simulink model "external_state_machine"  (R2021a)
settings: Solver=FixedStepDiscrete  StartTime=0.0  StopTime=3*t_ADC  RelTol=1e-3
values from neighbouring files (symbols this model uses):
  t_ADC = 1/f_ADC    (= 1e-05)    [uz_6ph_pu_vsd_voltages_init.m]    (also in uz_mpc_6ph_init.m; uz_mpc_6ph_state_machine_init.m; uz_typeconv_init.m)
  t_clock = 1/f_clock    (= 1e-08)    [uz_6ph_pu_vsd_voltages_init.m]    (also in uz_mpc_6ph_init.m; uz_mpc_6ph_state_machine_init.m; uz_typeconv_init.m)
libraries: simulink x5, hdlsllib x1
settings Model: DataTypeOverride=Off  Creator=micha  LastModifiedBy=micha
settings SolverCC: AlgebraicLoopSolver=TrustRegion
settings DataIOCC: LimitDataPoints=on  SaveOutput=off  SaveTime=off
settings OptimizationCC: BlockReduction=off  ConditionallyExecuteInputs=off  DefaultParameterBehavior=Inlined  LifeSpan=inf
settings DebuggingCC: AlgebraicLoopMsg=error  SingleTaskRateTransMsg=error  AllowSymbolicDim=off  StrictBusMsg=ErrorOnBusTreatedAsVector  SFUnexpectedBacktrackingDiag=warning  SFNoUnconditionalDefaultTransitionDiag=warning  SFExecutionAtInitializationDiag=none  SFMachineParentedDataDiag=warning  ArithmeticOperatorsInVariantConditions=warning
settings HardwareCC: ProdBitPerPointer=32  ProdBitPerSizeT=32  ProdBitPerPtrDiffT=32  ProdLargestAtomicFloat=None  ProdIntDivRoundTo=Undefined  ProdEndianess=Unspecified  ProdWordSize=32  ProdHWDeviceType=ASIC/FPGA->ASIC/FPGA  ProdEqTarget=off
settings SFSimCC: SimUseLocalCustomCode=off  CustomCodeUndefinedFunction=UseInterfaceOnly
settings RTWCC: RTWUseLocalCustomCode=off
settings CodeAppCC: StateflowObjectComments=on
settings GRTTargetCC: TargetLangStandard=C89/C90 (ANSI)
settings ConfigComp: CovScope=ReferencedModels  CovMetricSettings=dw  CovSaveCumulativeToWorkspaceVar=on  CovSaveSingleToWorkspaceVar=on  CovExternalEMLEnable=off  CovSFcnEnable=off

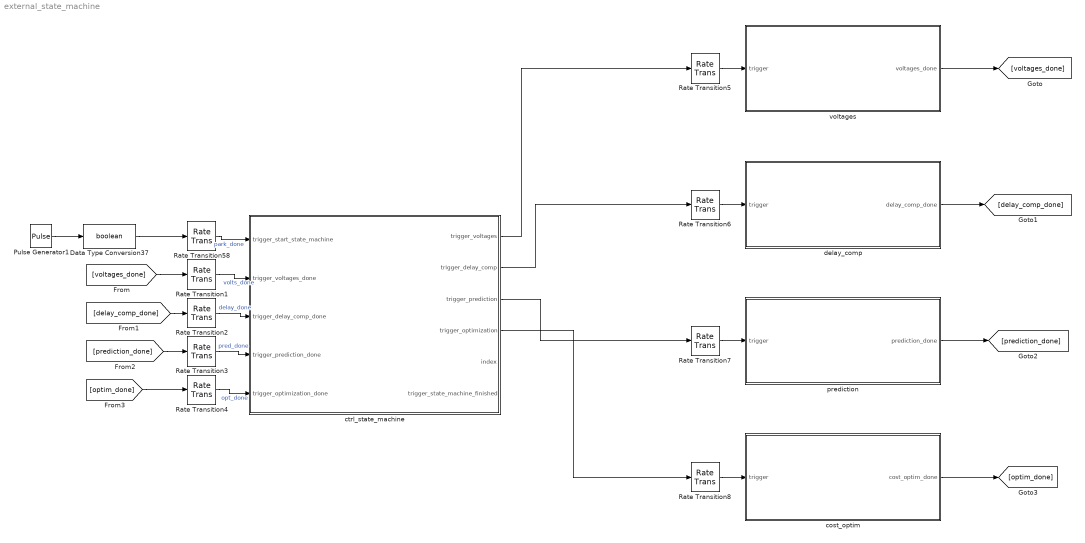
== system external_state_machine ==
  Data Type Conversion37 : DataTypeConversion  OutDataTypeStr=boolean
  Pulse Generator1 : DiscretePulseGenerator  PulseType=Time based  Period=t_ADC  PulseWidth=5
  Rate Transition{1..8,58} (9 alike) : RateTransition  OutPortSampleTime=t_clock
  cost_optim : Subsystem
  ctrl_state_machine : Subsystem
  delay_comp : Subsystem
  prediction : Subsystem
  voltages : Subsystem
  wires:
  ctrl_state_machine/2(trigger_delay_comp) -> Rate Transition6/1
  ctrl_state_machine/3(trigger_prediction) -> Rate Transition7/1
  ctrl_state_machine/4(trigger_optimization) -> Rate Transition8/1
  voltages/1(voltages_done) -> [voltages_done]
  delay_comp/1(delay_comp_done) -> [delay_comp_done]
  prediction/1(prediction_done) -> [prediction_done]
  cost_optim/1(cost_optim_done) -> [optim_done]
  [optim_done] -> Rate Transition4/1
  [prediction_done] -> Rate Transition3/1
  [delay_comp_done] -> Rate Transition2/1
  [voltages_done] -> Rate Transition1/1
  Data Type Conversion37/1 -> Rate Transition58/1
  Rate Transition58/1 -> ctrl_state_machine/1(trigger_start_state_machine)  "park_done"
  Pulse Generator1/1 -> Data Type Conversion37/1
  Rate Transition1/1 -> ctrl_state_machine/2(trigger_voltages_done)  "volts_done"
  Rate Transition2/1 -> ctrl_state_machine/3(trigger_delay_comp_done)  "delay_done"
  Rate Transition3/1 -> ctrl_state_machine/4(trigger_prediction_done)  "pred_done"
  Rate Transition4/1 -> ctrl_state_machine/5(trigger_optimization_done)  "opt_done"
  Rate Transition5/1 -> voltages/1(trigger)
  Rate Transition6/1 -> delay_comp/1(trigger)
  Rate Transition7/1 -> prediction/1(trigger)
  Rate Transition8/1 -> cost_optim/1(trigger)
  ctrl_state_machine/1(trigger_voltages) -> Rate Transition5/1

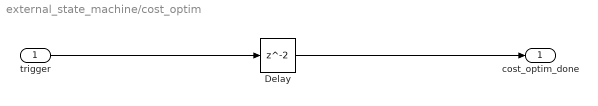
== system external_state_machine/cost_optim ==
  trigger : Inport
  Delay : Delay
  cost_optim_done : Outport  VectorParamsAs1DForOutWhenUnconnected=off
  wires:
  trigger/1 -> Delay/1
  Delay/1 -> cost_optim_done/1

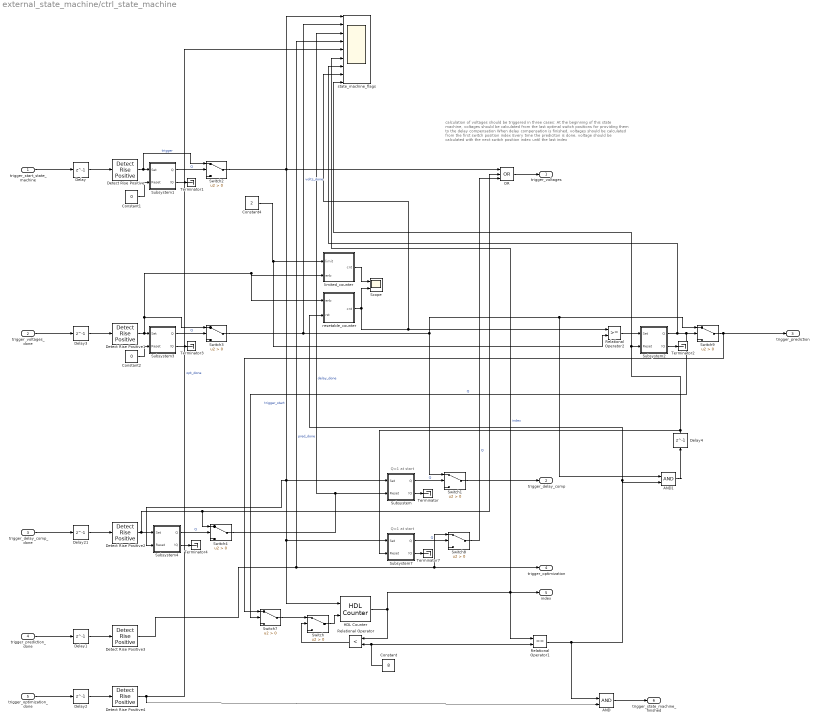
== system external_state_machine/ctrl_state_machine ==
  note: calculation of voltages should be triggered in three cases:
      |
      | At the beginning of this state machine, voltages should be calculated from the last optimal switch positions for providing them to the delay compensation
      | When delay compensation is finished, voltages should be calculated from the first switch position index
      | Every time the prediciton is done, voltage should be calculated with the next switch position index until the last index
  note: Q=1 at start
  note: Q=1 at start
  trigger_start_state_machine : Inport
  trigger_voltages_done : Inport  Port=2
  trigger_delay_comp_done : Inport  Port=3
  trigger_prediction_done : Inport  Port=4
  trigger_optimization_done : Inport  Port=5
  AND : Logic  IconShape=distinctive  AllPortsSameDT=off  OutDataTypeStr=boolean
  AND1 : Logic  IconShape=distinctive  AllPortsSameDT=off  OutDataTypeStr=boolean
  Constant : Constant  Value=8  OutDataTypeStr=uint32  SampleTime=-1
  Constant1 : Constant  Value=0  OutDataTypeStr=boolean  SampleTime=-1
  Constant2 : Constant  Value=0  OutDataTypeStr=boolean  SampleTime=-1
  Constant4 : Constant  Value=2  OutDataTypeStr=uint8  SampleTime=-1
  Delay{,1..4,21} (6 alike) : Delay  DelayLength=1
  Detect Rise Positive{,1..4} (5 alike) : simulink/Logic and Bit Operations/Detect Rise Positive  vinit=0  OutDataTypeStr=boolean
  HDL Counter : hdlsllib/Sources/HDL Counter  CountType=Free running  CountInit=1  CountStep=1  CountMax=25  CountFromType=Initial value  CountFrom=1  CountResetPort=on  CountLoadPort=off  CountEnbPort=on  CountDirPort=off  CountHitOutputPort=off  CountDataType=Unsigned  CountWordLen=32  CountFracLen=0  CountSampTime=1
  OR : Logic  Operator=OR  Inputs=3  IconShape=distinctive  AllPortsSameDT=off  OutDataTypeStr=boolean
  Relational Operator : RelationalOperator  Operator=<  OutDataTypeStr=boolean  RndMeth=Simplest
  Relational Operator1 : RelationalOperator  Operator===  OutDataTypeStr=boolean  RndMeth=Simplest
  Relational Operator2 : RelationalOperator  OutDataTypeStr=boolean  RndMeth=Simplest
  Scope : Scope  NumInputPorts=2
  Subsystem : Subsystem
  Subsystem1 : Subsystem
  Subsystem2 : Subsystem
  Subsystem3 : Subsystem
  Subsystem4 : Subsystem
  Subsystem7 : Subsystem
  Switch{,1..4,7..9} (8 alike) : Switch  Criteria=u2 > Threshold
  Terminator{,1..4,7} (6 alike) : Terminator
  limited_counter : Subsystem
  resetable_counter : Subsystem
  state_machine_flags : Scope  NumInputPorts=9
  trigger_voltages : Outport  VectorParamsAs1DForOutWhenUnconnected=off
  trigger_delay_comp : Outport  Port=2  VectorParamsAs1DForOutWhenUnconnected=off
  trigger_prediction : Outport  Port=3  VectorParamsAs1DForOutWhenUnconnected=off
  trigger_optimization : Outport  Port=4  VectorParamsAs1DForOutWhenUnconnected=off
  index : Outport  Port=5  VectorParamsAs1DForOutWhenUnconnected=off
  trigger_state_machine_finished : Outport  Port=6  VectorParamsAs1DForOutWhenUnconnected=off
  wires:
  OR/1 -> trigger_voltages/1
  Constant/1 -> Relational Operator/2, Relational Operator1/2
  Relational Operator/1 -> Switch/2
  Switch2/1 -> state_machine_flags/1, HDL Counter/1, Subsystem7/1(Set), Subsystem/1(Set), Subsystem4/2(Reset), OR/1  "trigger_start"
  Subsystem/1(Q) -> Switch1/2  "Q"
  Subsystem/2(!Q) -> Terminator/1
  Switch1/1 -> trigger_delay_comp/1
  Subsystem1/2(!Q) -> Terminator1/1
  Subsystem1/1(Q) -> Switch2/2  "Q"
  trigger_voltages_done/1 -> Delay3/1
  trigger_delay_comp_done/1 -> Delay21/1
  Delay21/1 -> Detect Rise Positive2/1
  Delay/1 -> Detect Rise Positive/1
  trigger_start_state_machine/1 -> Delay/1
  Delay2/1 -> Detect Rise Positive4/1
  trigger_optimization_done/1 -> Delay2/1
  Delay1/1 -> Detect Rise Positive3/1
  trigger_prediction_done/1 -> Delay1/1
  Detect Rise Positive/1 -> Switch2/1, Subsystem1/1(Set)  "trigger"
  Subsystem3/1(Q) -> Switch3/2  "Q"
  Subsystem3/2(!Q) -> Terminator3/1
  Subsystem4/1(Q) -> Switch4/2  "Q"
  Subsystem4/2(!Q) -> Terminator4/1
  Detect Rise Positive2/1 -> OR/2, Switch4/1, Subsystem4/1(Set)
  Switch4/1 -> state_machine_flags/3, Subsystem/2(Reset)  "delay_done"
  Constant1/1 -> Subsystem1/2(Reset)
  Constant2/1 -> Subsystem3/2(Reset)
  Detect Rise Positive1/1 -> resetable_counter/1(enb), limited_counter/2(enb), Switch3/1, Subsystem3/1(Set)
  Switch3/1 -> state_machine_flags/2, AND1/1, Switch9/1, Switch1/1  "volts_done"
  Delay3/1 -> Detect Rise Positive1/1
  Subsystem2/2(!Q) -> Terminator2/1
  Subsystem2/1(Q) -> state_machine_flags/7, Switch7/2, Switch9/2  "Q"
  Constant4/1 -> Relational Operator2/2, limited_counter/1(limit)
  Relational Operator2/1 -> Subsystem2/1(Set)
  limited_counter/1(cnt) -> Scope/1
  Detect Rise Positive3/1 -> state_machine_flags/4, Switch8/1, trigger_optimization/1  "pred_done"
  Switch/1 -> HDL Counter/2
  HDL Counter/1 -> Relational Operator1/1, state_machine_flags/6, index/1, Relational Operator/1  "index"
  Detect Rise Positive4/1 -> state_machine_flags/5, AND/2  "opt_done"
  Switch7/1 -> Switch/1
  resetable_counter/1(cnt) -> Scope/2, state_machine_flags/8, Relational Operator2/1
  Relational Operator1/1 -> AND1/2, resetable_counter/2(rst), AND/1
  Switch9/1 -> Switch7/1, trigger_prediction/1
  AND/1 -> trigger_state_machine_finished/1
  AND1/1 -> Delay4/1
  Delay4/1 -> state_machine_flags/9, Subsystem2/2(Reset), Subsystem7/2(Reset)
  Switch8/1 -> OR/3  "Q"
  Subsystem7/2(!Q) -> Terminator7/1
  Subsystem7/1(Q) -> Switch8/2  "Q"

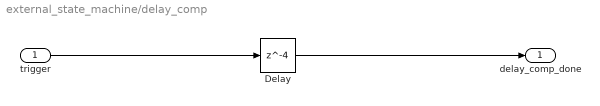
== system external_state_machine/delay_comp ==
  trigger : Inport
  Delay : Delay  DelayLength=4
  delay_comp_done : Outport  VectorParamsAs1DForOutWhenUnconnected=off
  wires:
  trigger/1 -> Delay/1
  Delay/1 -> delay_comp_done/1

== system external_state_machine/prediction ==
  trigger : Inport
  Delay : Delay  DelayLength=5
  prediction_done : Outport  VectorParamsAs1DForOutWhenUnconnected=off
  wires:
  trigger/1 -> Delay/1
  Delay/1 -> prediction_done/1

== system external_state_machine/voltages ==
  trigger : Inport
  Delay : Delay  DelayLength=4
  voltages_done : Outport  VectorParamsAs1DForOutWhenUnconnected=off
  wires:
  trigger/1 -> Delay/1
  Delay/1 -> voltages_done/1

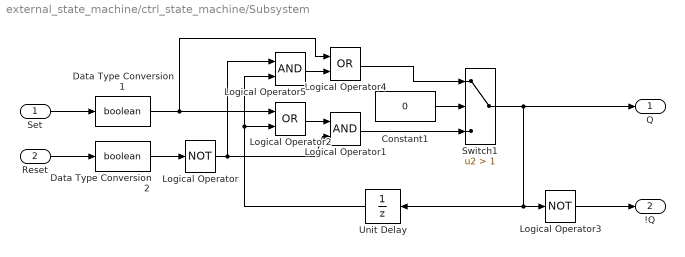
== system external_state_machine/ctrl_state_machine/Subsystem ==
  Set : Inport
  Reset : Inport  Port=2
  Constant1 : Constant  Value=0  OutDataTypeStr=uint32  SampleTime=-1
  Data Type Conversion1 : DataTypeConversion  OutDataTypeStr=boolean
  Data Type Conversion2 : DataTypeConversion  OutDataTypeStr=boolean
  Logical Operator : Logic  Operator=NOT  AllPortsSameDT=off  OutDataTypeStr=boolean
  Logical Operator1 : Logic  AllPortsSameDT=off  OutDataTypeStr=boolean
  Logical Operator2 : Logic  Operator=OR  AllPortsSameDT=off  OutDataTypeStr=boolean
  Logical Operator3 : Logic  Operator=NOT  AllPortsSameDT=off  OutDataTypeStr=boolean
  Logical Operator4 : Logic  Operator=OR  AllPortsSameDT=off  OutDataTypeStr=boolean
  Logical Operator5 : Logic  AllPortsSameDT=off  OutDataTypeStr=boolean
  Switch1 : Switch  Criteria=u2 > Threshold  Threshold=1
  Unit Delay : UnitDelay  InitialCondition=1  SampleTime=t_clock  HasFrameUpgradeWarning=on
  Q : Outport  VectorParamsAs1DForOutWhenUnconnected=off
  !Q : Outport  Port=2  VectorParamsAs1DForOutWhenUnconnected=off
  wires:
  Logical Operator/1 -> Logical Operator1/2, Logical Operator5/1
  Reset/1 -> Data Type Conversion2/1
  Constant1/1 -> Switch1/2
  Logical Operator4/1 -> Switch1/1
  Data Type Conversion1/1 -> Logical Operator2/1, Logical Operator4/1
  Switch1/1 -> Q/1, Unit Delay/1, Logical Operator3/1
  Logical Operator3/1 -> !Q/1
  Set/1 -> Data Type Conversion1/1
  Logical Operator2/1 -> Logical Operator1/1
  Unit Delay/1 -> Logical Operator2/2, Logical Operator5/2
  Logical Operator5/1 -> Logical Operator4/2
  Logical Operator1/1 -> Switch1/3
  Data Type Conversion2/1 -> Logical Operator/1

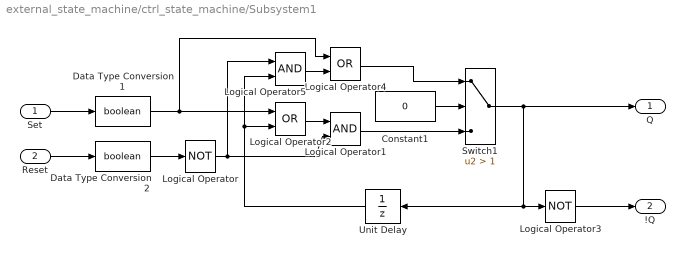
== system external_state_machine/ctrl_state_machine/Subsystem1 ==
  Set : Inport
  Reset : Inport  Port=2
  Constant1 : Constant  Value=0  OutDataTypeStr=uint32  SampleTime=-1
  Data Type Conversion1 : DataTypeConversion  OutDataTypeStr=boolean
  Data Type Conversion2 : DataTypeConversion  OutDataTypeStr=boolean
  Logical Operator : Logic  Operator=NOT  AllPortsSameDT=off  OutDataTypeStr=boolean
  Logical Operator1 : Logic  AllPortsSameDT=off  OutDataTypeStr=boolean
  Logical Operator2 : Logic  Operator=OR  AllPortsSameDT=off  OutDataTypeStr=boolean
  Logical Operator3 : Logic  Operator=NOT  AllPortsSameDT=off  OutDataTypeStr=boolean
  Logical Operator4 : Logic  Operator=OR  AllPortsSameDT=off  OutDataTypeStr=boolean
  Logical Operator5 : Logic  AllPortsSameDT=off  OutDataTypeStr=boolean
  Switch1 : Switch  Criteria=u2 > Threshold  Threshold=1
  Unit Delay : UnitDelay  SampleTime=t_clock  HasFrameUpgradeWarning=on
  Q : Outport  VectorParamsAs1DForOutWhenUnconnected=off
  !Q : Outport  Port=2  VectorParamsAs1DForOutWhenUnconnected=off
  wires:
  Logical Operator/1 -> Logical Operator1/2, Logical Operator5/1
  Reset/1 -> Data Type Conversion2/1
  Constant1/1 -> Switch1/2
  Logical Operator4/1 -> Switch1/1
  Data Type Conversion1/1 -> Logical Operator2/1, Logical Operator4/1
  Switch1/1 -> Q/1, Unit Delay/1, Logical Operator3/1
  Logical Operator3/1 -> !Q/1
  Set/1 -> Data Type Conversion1/1
  Logical Operator2/1 -> Logical Operator1/1
  Unit Delay/1 -> Logical Operator2/2, Logical Operator5/2
  Logical Operator5/1 -> Logical Operator4/2
  Logical Operator1/1 -> Switch1/3
  Data Type Conversion2/1 -> Logical Operator/1

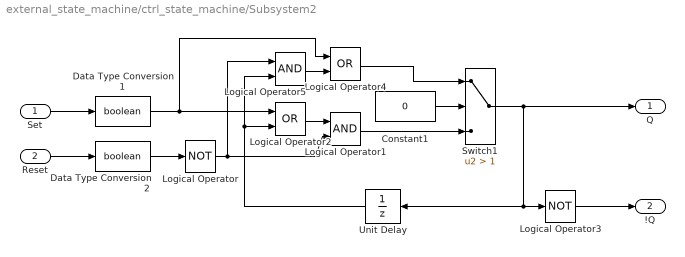
== system external_state_machine/ctrl_state_machine/Subsystem2 ==
  Set : Inport
  Reset : Inport  Port=2
  Constant1 : Constant  Value=0  OutDataTypeStr=uint32  SampleTime=-1
  Data Type Conversion1 : DataTypeConversion  OutDataTypeStr=boolean
  Data Type Conversion2 : DataTypeConversion  OutDataTypeStr=boolean
  Logical Operator : Logic  Operator=NOT  AllPortsSameDT=off  OutDataTypeStr=boolean
  Logical Operator1 : Logic  AllPortsSameDT=off  OutDataTypeStr=boolean
  Logical Operator2 : Logic  Operator=OR  AllPortsSameDT=off  OutDataTypeStr=boolean
  Logical Operator3 : Logic  Operator=NOT  AllPortsSameDT=off  OutDataTypeStr=boolean
  Logical Operator4 : Logic  Operator=OR  AllPortsSameDT=off  OutDataTypeStr=boolean
  Logical Operator5 : Logic  AllPortsSameDT=off  OutDataTypeStr=boolean
  Switch1 : Switch  Criteria=u2 > Threshold  Threshold=1
  Unit Delay : UnitDelay  SampleTime=t_clock  HasFrameUpgradeWarning=on
  Q : Outport  VectorParamsAs1DForOutWhenUnconnected=off
  !Q : Outport  Port=2  VectorParamsAs1DForOutWhenUnconnected=off
  wires:
  Logical Operator/1 -> Logical Operator1/2, Logical Operator5/1
  Reset/1 -> Data Type Conversion2/1
  Constant1/1 -> Switch1/2
  Logical Operator4/1 -> Switch1/1
  Data Type Conversion1/1 -> Logical Operator2/1, Logical Operator4/1
  Switch1/1 -> Q/1, Unit Delay/1, Logical Operator3/1
  Logical Operator3/1 -> !Q/1
  Set/1 -> Data Type Conversion1/1
  Logical Operator2/1 -> Logical Operator1/1
  Unit Delay/1 -> Logical Operator2/2, Logical Operator5/2
  Logical Operator5/1 -> Logical Operator4/2
  Logical Operator1/1 -> Switch1/3
  Data Type Conversion2/1 -> Logical Operator/1

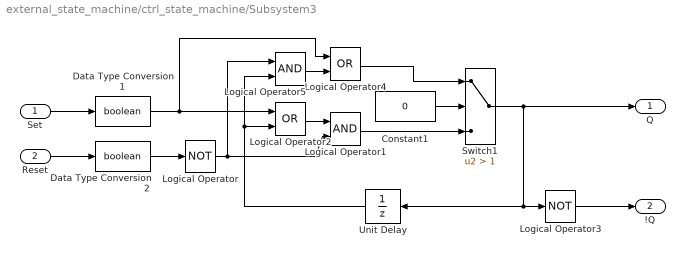
== system external_state_machine/ctrl_state_machine/Subsystem3 ==
  Set : Inport
  Reset : Inport  Port=2
  Constant1 : Constant  Value=0  OutDataTypeStr=uint32  SampleTime=-1
  Data Type Conversion1 : DataTypeConversion  OutDataTypeStr=boolean
  Data Type Conversion2 : DataTypeConversion  OutDataTypeStr=boolean
  Logical Operator : Logic  Operator=NOT  AllPortsSameDT=off  OutDataTypeStr=boolean
  Logical Operator1 : Logic  AllPortsSameDT=off  OutDataTypeStr=boolean
  Logical Operator2 : Logic  Operator=OR  AllPortsSameDT=off  OutDataTypeStr=boolean
  Logical Operator3 : Logic  Operator=NOT  AllPortsSameDT=off  OutDataTypeStr=boolean
  Logical Operator4 : Logic  Operator=OR  AllPortsSameDT=off  OutDataTypeStr=boolean
  Logical Operator5 : Logic  AllPortsSameDT=off  OutDataTypeStr=boolean
  Switch1 : Switch  Criteria=u2 > Threshold  Threshold=1
  Unit Delay : UnitDelay  SampleTime=t_clock  HasFrameUpgradeWarning=on
  Q : Outport  VectorParamsAs1DForOutWhenUnconnected=off
  !Q : Outport  Port=2  VectorParamsAs1DForOutWhenUnconnected=off
  wires:
  Logical Operator/1 -> Logical Operator1/2, Logical Operator5/1
  Reset/1 -> Data Type Conversion2/1
  Constant1/1 -> Switch1/2
  Logical Operator4/1 -> Switch1/1
  Data Type Conversion1/1 -> Logical Operator2/1, Logical Operator4/1
  Switch1/1 -> Q/1, Unit Delay/1, Logical Operator3/1
  Logical Operator3/1 -> !Q/1
  Set/1 -> Data Type Conversion1/1
  Logical Operator2/1 -> Logical Operator1/1
  Unit Delay/1 -> Logical Operator2/2, Logical Operator5/2
  Logical Operator5/1 -> Logical Operator4/2
  Logical Operator1/1 -> Switch1/3
  Data Type Conversion2/1 -> Logical Operator/1

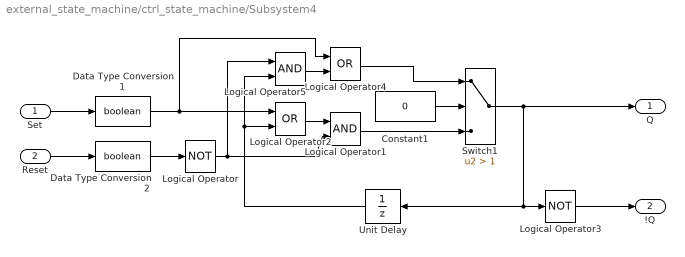
== system external_state_machine/ctrl_state_machine/Subsystem4 ==
  Set : Inport
  Reset : Inport  Port=2
  Constant1 : Constant  Value=0  OutDataTypeStr=uint32  SampleTime=-1
  Data Type Conversion1 : DataTypeConversion  OutDataTypeStr=boolean
  Data Type Conversion2 : DataTypeConversion  OutDataTypeStr=boolean
  Logical Operator : Logic  Operator=NOT  AllPortsSameDT=off  OutDataTypeStr=boolean
  Logical Operator1 : Logic  AllPortsSameDT=off  OutDataTypeStr=boolean
  Logical Operator2 : Logic  Operator=OR  AllPortsSameDT=off  OutDataTypeStr=boolean
  Logical Operator3 : Logic  Operator=NOT  AllPortsSameDT=off  OutDataTypeStr=boolean
  Logical Operator4 : Logic  Operator=OR  AllPortsSameDT=off  OutDataTypeStr=boolean
  Logical Operator5 : Logic  AllPortsSameDT=off  OutDataTypeStr=boolean
  Switch1 : Switch  Criteria=u2 > Threshold  Threshold=1
  Unit Delay : UnitDelay  SampleTime=t_clock  HasFrameUpgradeWarning=on
  Q : Outport  VectorParamsAs1DForOutWhenUnconnected=off
  !Q : Outport  Port=2  VectorParamsAs1DForOutWhenUnconnected=off
  wires:
  Logical Operator/1 -> Logical Operator1/2, Logical Operator5/1
  Reset/1 -> Data Type Conversion2/1
  Constant1/1 -> Switch1/2
  Logical Operator4/1 -> Switch1/1
  Data Type Conversion1/1 -> Logical Operator2/1, Logical Operator4/1
  Switch1/1 -> Q/1, Unit Delay/1, Logical Operator3/1
  Logical Operator3/1 -> !Q/1
  Set/1 -> Data Type Conversion1/1
  Logical Operator2/1 -> Logical Operator1/1
  Unit Delay/1 -> Logical Operator2/2, Logical Operator5/2
  Logical Operator5/1 -> Logical Operator4/2
  Logical Operator1/1 -> Switch1/3
  Data Type Conversion2/1 -> Logical Operator/1

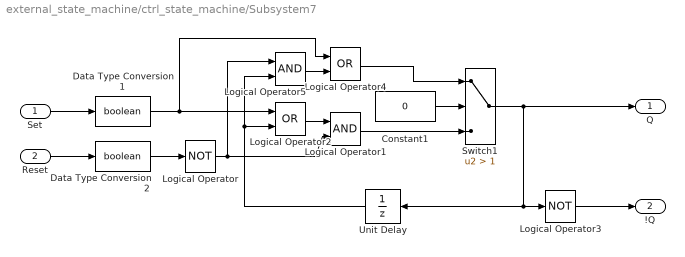
== system external_state_machine/ctrl_state_machine/Subsystem7 ==
  Set : Inport
  Reset : Inport  Port=2
  Constant1 : Constant  Value=0  OutDataTypeStr=uint32  SampleTime=-1
  Data Type Conversion1 : DataTypeConversion  OutDataTypeStr=boolean
  Data Type Conversion2 : DataTypeConversion  OutDataTypeStr=boolean
  Logical Operator : Logic  Operator=NOT  AllPortsSameDT=off  OutDataTypeStr=boolean
  Logical Operator1 : Logic  AllPortsSameDT=off  OutDataTypeStr=boolean
  Logical Operator2 : Logic  Operator=OR  AllPortsSameDT=off  OutDataTypeStr=boolean
  Logical Operator3 : Logic  Operator=NOT  AllPortsSameDT=off  OutDataTypeStr=boolean
  Logical Operator4 : Logic  Operator=OR  AllPortsSameDT=off  OutDataTypeStr=boolean
  Logical Operator5 : Logic  AllPortsSameDT=off  OutDataTypeStr=boolean
  Switch1 : Switch  Criteria=u2 > Threshold  Threshold=1
  Unit Delay : UnitDelay  InitialCondition=1  SampleTime=t_clock  HasFrameUpgradeWarning=on
  Q : Outport  VectorParamsAs1DForOutWhenUnconnected=off
  !Q : Outport  Port=2  VectorParamsAs1DForOutWhenUnconnected=off
  wires:
  Logical Operator/1 -> Logical Operator1/2, Logical Operator5/1
  Reset/1 -> Data Type Conversion2/1
  Constant1/1 -> Switch1/2
  Logical Operator4/1 -> Switch1/1
  Data Type Conversion1/1 -> Logical Operator2/1, Logical Operator4/1
  Switch1/1 -> Q/1, Unit Delay/1, Logical Operator3/1
  Logical Operator3/1 -> !Q/1
  Set/1 -> Data Type Conversion1/1
  Logical Operator2/1 -> Logical Operator1/1
  Unit Delay/1 -> Logical Operator2/2, Logical Operator5/2
  Logical Operator5/1 -> Logical Operator4/2
  Logical Operator1/1 -> Switch1/3
  Data Type Conversion2/1 -> Logical Operator/1

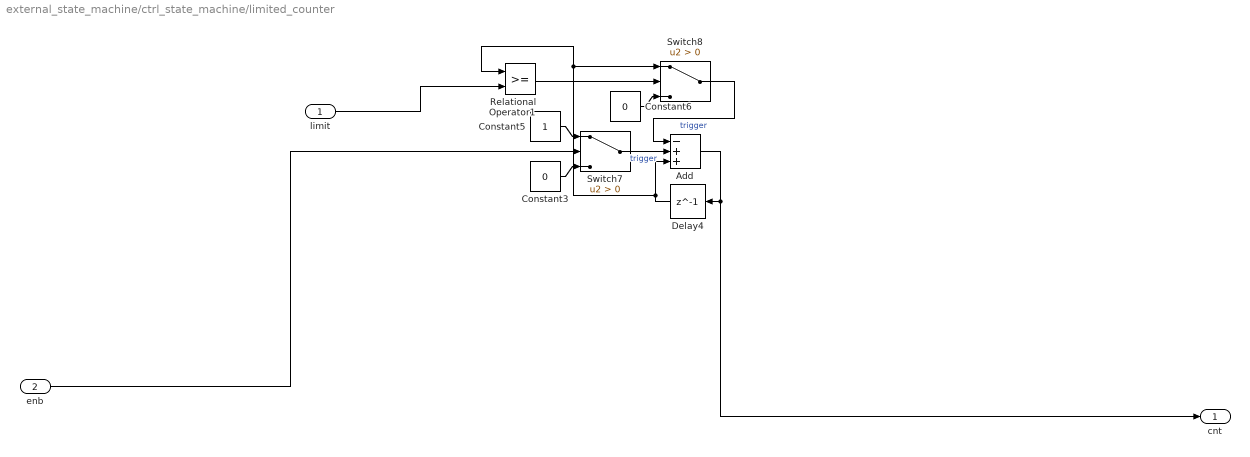
== system external_state_machine/ctrl_state_machine/limited_counter ==
  limit : Inport
  enb : Inport  Port=2
  Add : Sum  Inputs=-++  AccumDataTypeStr=uint8
  Constant3 : Constant  Value=0  OutDataTypeStr=uint8  SampleTime=-1
  Constant5 : Constant  OutDataTypeStr=uint8  SampleTime=-1
  Constant6 : Constant  Value=0  OutDataTypeStr=uint8  SampleTime=-1
  Delay4 : Delay  DelayLength=1
  Relational Operator1 : RelationalOperator  OutDataTypeStr=boolean  RndMeth=Simplest
  Switch7 : Switch  Criteria=u2 > Threshold
  Switch8 : Switch  Criteria=u2 > Threshold
  cnt : Outport
  wires:
  Constant6/1 -> Switch8/3
  Constant3/1 -> Switch7/3
  Switch8/1 -> Add/1  "trigger"
  Delay4/1 -> Add/3, Relational Operator1/1, Switch8/1
  Switch7/1 -> Add/2  "trigger"
  Constant5/1 -> Switch7/1
  Relational Operator1/1 -> Switch8/2
  Add/1 -> cnt/1, Delay4/1
  limit/1 -> Relational Operator1/2
  enb/1 -> Switch7/2

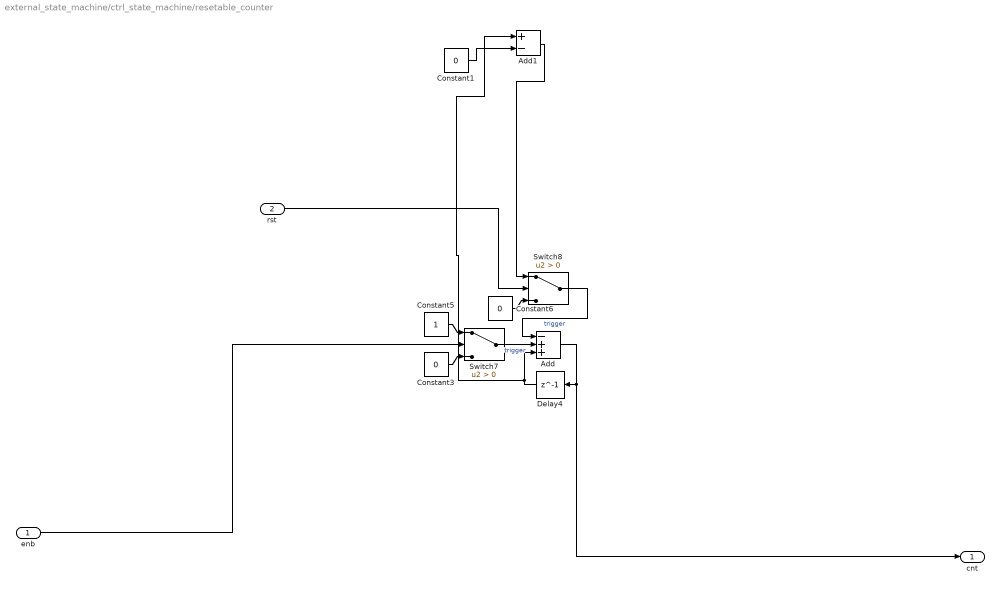
== system external_state_machine/ctrl_state_machine/resetable_counter ==
  enb : Inport
  rst : Inport  Port=2
  Add : Sum  Inputs=-++  AccumDataTypeStr=uint8
  Add1 : Sum  Inputs=+-  AccumDataTypeStr=uint8
  Constant1 : Constant  Value=0  OutDataTypeStr=uint8  SampleTime=-1
  Constant3 : Constant  Value=0  OutDataTypeStr=uint8  SampleTime=-1
  Constant5 : Constant  OutDataTypeStr=uint8  SampleTime=-1
  Constant6 : Constant  Value=0  OutDataTypeStr=uint8  SampleTime=-1
  Delay4 : Delay  DelayLength=1
  Switch7 : Switch  Criteria=u2 > Threshold
  Switch8 : Switch  Criteria=u2 > Threshold
  cnt : Outport
  wires:
  Constant6/1 -> Switch8/3
  Constant3/1 -> Switch7/3
  Switch8/1 -> Add/1  "trigger"
  Switch7/1 -> Add/2  "trigger"
  Constant5/1 -> Switch7/1
  Add/1 -> cnt/1, Delay4/1
  enb/1 -> Switch7/2
  Constant1/1 -> Add1/2
  Add1/1 -> Switch8/1
  Delay4/1 -> Add/3, Add1/1
  rst/1 -> Switch8/2
